simulink model "audio_tone"  (R2018b)
settings: Solver=FixedStepAuto  StartTime=0.0  StopTime=0.2  RelTol=1e-3
libraries: hdlsllib x1
settings Model: Creator=caeuser  LastModifiedBy=caeuser
settings OptimizationCC: BlockReduction=off  ConditionallyExecuteInputs=off  DefaultParameterBehavior=Inlined
settings DebuggingCC: AlgebraicLoopMsg=error
settings HardwareCC: ProdBitPerPointer=32  ProdBitPerSizeT=32  ProdBitPerPtrDiffT=32  ProdLargestAtomicFloat=None  ProdIntDivRoundTo=Undefined  ProdEndianess=Unspecified  ProdWordSize=32  ProdHWDeviceType=ASIC/FPGA->ASIC/FPGA  TargetBitPerLong=64  TargetBitPerPointer=64  TargetBitPerSizeT=64  TargetBitPerPtrDiffT=64  TargetLongLongMode=on  TargetIntDivRoundTo=Zero  TargetEndianess=LittleEndian  TargetWordSize=64  TargetHWDeviceType=Custom Processor->MATLAB Host Computer  ProdEqTarget=off

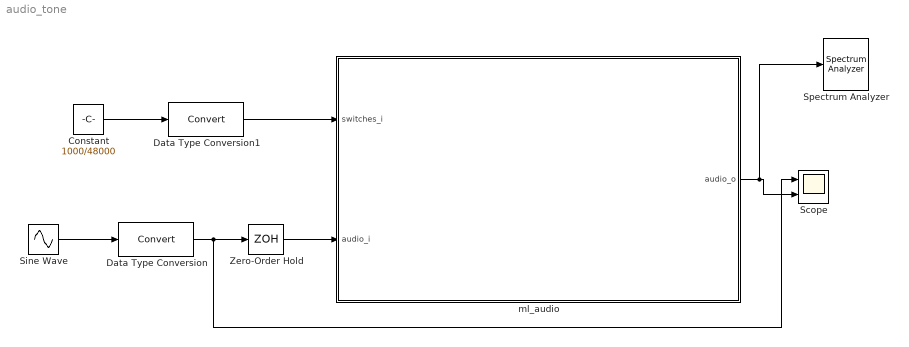
== system audio_tone ==
  Constant : Constant  Value=1000/48000  SampleTime=1/48000
  Data Type Conversion : DataTypeConversion
  Data Type Conversion1 : DataTypeConversion  SaturateOnIntegerOverflow=on
  Scope : Scope  NumInputPorts=2
  Sine Wave : Sin  Amplitude=0.1  Frequency=2*3.14*30  SampleTime=0
  Spectrum Analyzer : SpectrumAnalyzer
  Zero-Order Hold : ZeroOrderHold  SampleTime=1/48000
  ml_audio : Subsystem
  wires:
  Constant/1 -> Data Type Conversion1/1
  Data Type Conversion/1 -> Zero-Order Hold/1, Scope/1
  Data Type Conversion1/1 -> ml_audio/1(switches_i)
  ml_audio/1(audio_o) -> Spectrum Analyzer/1, Scope/2
  Zero-Order Hold/1 -> ml_audio/2(audio_i)
  Sine Wave/1 -> Data Type Conversion/1

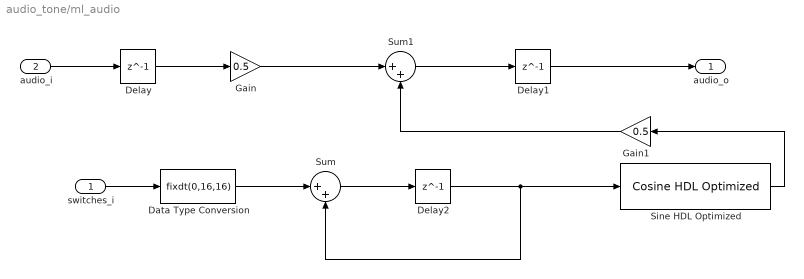
== system audio_tone/ml_audio ==
  switches_i : Inport  OutDataTypeStr=fixdt(0,10,10)
  audio_i : Inport  Port=2  OutDataTypeStr=fixdt(1,16,15)
  Data Type Conversion : DataTypeConversion  OutDataTypeStr=fixdt(0,16,16)
  Delay : Delay  DelayLength=1  InitialCondition=0
  Delay1 : Delay  DelayLength=1  InitialCondition=0
  Delay2 : Delay  DelayLength=1  InitialCondition=0
  Gain : Gain  Gain=0.5  OutDataTypeStr=Inherit: Same as input
  Gain1 : Gain  Gain=0.5  OutDataTypeStr=fixdt(1,16,15)
  Sine HDL Optimized : hdlsllib/Lookup Tables/Cosine HDL Optimized  OutputFormula=sin(2*pi*u)  NumDataPoints=16384  TableDataTypeStr=fixdt(1,15,14)  SimulateLUTROMDelay=off
      settings: SourceProductName=HDL Coder  SourceProductBaseCode=HD
  Sum : Sum  Inputs=|++  AccumDataTypeStr=fixdt(0,16,16)
  Sum1 : Sum  Inputs=|++
  audio_o : Outport  OutDataTypeStr=fixdt(1,16,15)
  wires:
  audio_i/1 -> Delay/1
  Delay1/1 -> audio_o/1
  Delay2/1 -> Sine HDL Optimized/1, Sum/2
  Sum/1 -> Delay2/1
  Sine HDL Optimized/1 -> Gain1/1
  Sum1/1 -> Delay1/1
  switches_i/1 -> Data Type Conversion/1
  Data Type Conversion/1 -> Sum/1
  Delay/1 -> Gain/1
  Gain1/1 -> Sum1/2
  Gain/1 -> Sum1/1
